simulink model "F_S"  (R2013a)
settings: Solver=ode45  StartTime=0.0  StopTime=0.2  RelTol=1e-3
settings Model: Creator=MEHEDI HASSAN  LastModifiedBy=BORAT
settings OptimizationCC: InlineParams=on
settings DebuggingCC: SolverPrmCheckMsg=none  ModelReferenceExtraNoncontSigs=none

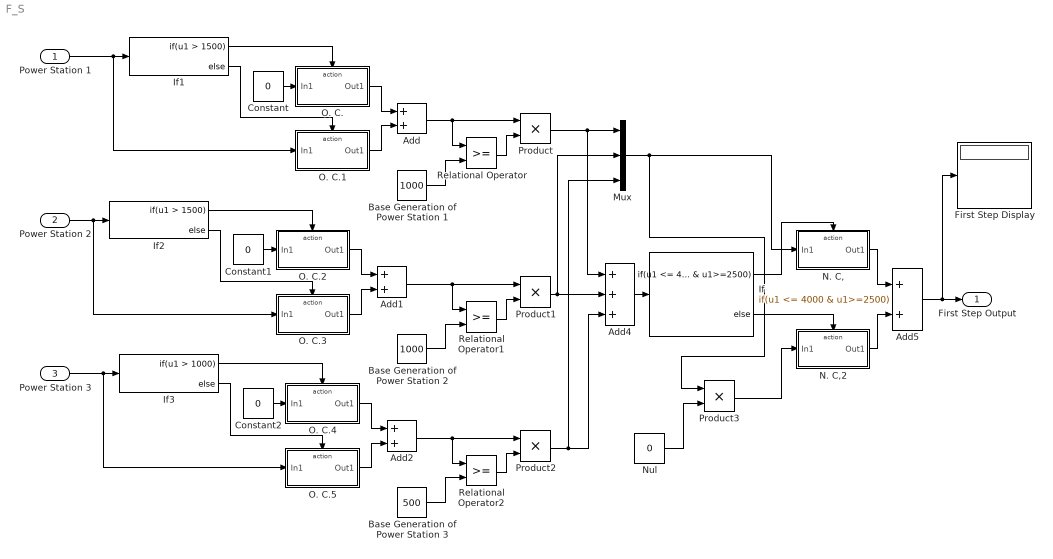
== system F_S ==
  Power Station 1 : Inport
  Power Station 2 : Inport  Port=2
  Power Station 3 : Inport  Port=3
  Add{,1..2,5} (4 alike) : Sum
  Add4 : Sum  Inputs=+++
  Base Generation of Power Station 1 : Constant  Value=1000
  Base Generation of Power Station 2 : Constant  Value=1000
  Base Generation of Power Station 3 : Constant  Value=500
  Constant : Constant  Value=0
  Constant1 : Constant  Value=0
  Constant2 : Constant  Value=0
  First Step Display : Display
  If : If  IfExpression=u1 <= 4000 & u1>=2500
  If1 : If  IfExpression=u1 > 1500
  If2 : If  IfExpression=u1 > 1500
  If3 : If  IfExpression=u1 > 1000
  Mux : Mux  Inputs=3
  N. C, : Subsystem  TreatAsAtomicUnit=on
  N. C,2 : Subsystem  TreatAsAtomicUnit=on
  Nul : Constant  Value=0
  O. C. : Subsystem  TreatAsAtomicUnit=on
  O. C.1 : Subsystem  TreatAsAtomicUnit=on
  O. C.2 : Subsystem  TreatAsAtomicUnit=on
  O. C.3 : Subsystem  TreatAsAtomicUnit=on
  O. C.4 : Subsystem  TreatAsAtomicUnit=on
  O. C.5 : Subsystem  TreatAsAtomicUnit=on
  Product{,1..3} (4 alike) : Product
  Relational Operator : RelationalOperator  OutDataTypeStr=boolean
  Relational Operator1 : RelationalOperator  OutDataTypeStr=boolean
  Relational Operator2 : RelationalOperator  OutDataTypeStr=boolean
  First Step Output : Outport
  wires:
  Base Generation of Power Station 1/1 -> Relational Operator/2
  Relational Operator/1 -> Product/2
  Base Generation of Power Station 2/1 -> Relational Operator1/2
  Relational Operator1/1 -> Product1/2
  Base Generation of Power Station 3/1 -> Relational Operator2/2
  Relational Operator2/1 -> Product2/2
  Product/1 -> Add4/1, Mux/1
  Product1/1 -> Mux/2, Add4/2
  Product2/1 -> Add4/3, Mux/3
  Add4/1 -> If/1
  If/2 -> N. C,2/Action
  Mux/1 -> N. C,/1(In1), Product3/1
  Product3/1 -> N. C,2/1(In1)
  Nul/1 -> Product3/2
  N. C,/1(Out1) -> Add5/1
  If/1 -> N. C,/Action
  Add5/1 -> First Step Output/1, First Step Display/1
  N. C,2/1(Out1) -> Add5/2
  Constant/1 -> O. C./1(In1)
  Power Station 1/1 -> O. C.1/1(In1), If1/1
  If1/1 -> O. C./Action
  If1/2 -> O. C.1/Action
  O. C./1(Out1) -> Add/1
  O. C.1/1(Out1) -> Add/2
  Add/1 -> Relational Operator/1, Product/1
  Constant1/1 -> O. C.2/1(In1)
  Power Station 2/1 -> O. C.3/1(In1), If2/1
  If2/1 -> O. C.2/Action
  If2/2 -> O. C.3/Action
  O. C.2/1(Out1) -> Add1/1
  O. C.3/1(Out1) -> Add1/2
  Add1/1 -> Relational Operator1/1, Product1/1
  Constant2/1 -> O. C.4/1(In1)
  Power Station 3/1 -> O. C.5/1(In1), If3/1
  If3/1 -> O. C.4/Action
  If3/2 -> O. C.5/Action
  O. C.4/1(Out1) -> Add2/1
  O. C.5/1(Out1) -> Add2/2
  Add2/1 -> Product2/1, Relational Operator2/1

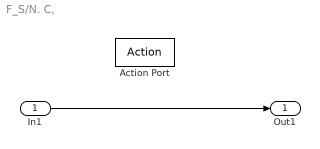
== system F_S/N. C, ==
  In1 : Inport
  Action Port : ActionPort  ActionType=then
  Out1 : Outport
  wires:
  In1/1 -> Out1/1

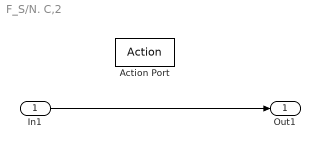
== system F_S/N. C,2 ==
  In1 : Inport
  Action Port : ActionPort  ActionType=else
  Out1 : Outport
  wires:
  In1/1 -> Out1/1

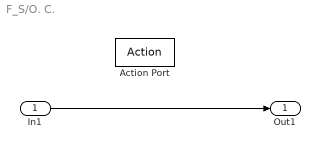
== system F_S/O. C. ==
  In1 : Inport
  Action Port : ActionPort  ActionType=then
  Out1 : Outport
  wires:
  In1/1 -> Out1/1

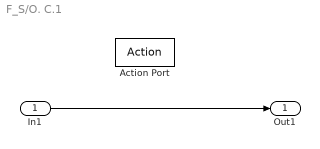
== system F_S/O. C.1 ==
  In1 : Inport
  Action Port : ActionPort  ActionType=else
  Out1 : Outport
  wires:
  In1/1 -> Out1/1

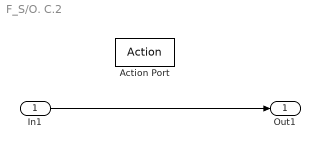
== system F_S/O. C.2 ==
  In1 : Inport
  Action Port : ActionPort  ActionType=then
  Out1 : Outport
  wires:
  In1/1 -> Out1/1

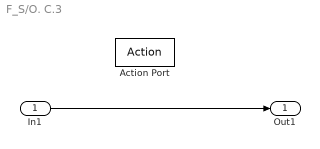
== system F_S/O. C.3 ==
  In1 : Inport
  Action Port : ActionPort  ActionType=else
  Out1 : Outport
  wires:
  In1/1 -> Out1/1

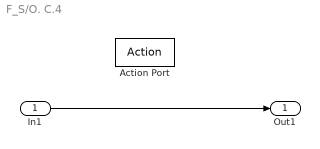
== system F_S/O. C.4 ==
  In1 : Inport
  Action Port : ActionPort  ActionType=then
  Out1 : Outport
  wires:
  In1/1 -> Out1/1

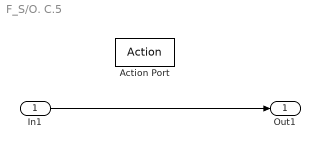
== system F_S/O. C.5 ==
  In1 : Inport
  Action Port : ActionPort  ActionType=else
  Out1 : Outport
  wires:
  In1/1 -> Out1/1
